simulink model "dc_motor"  (R2024a)
settings: Solver=VariableStepAuto  StartTime=0.0  StopTime=10.0  RelTol=1e-3
values from neighbouring files (symbols this model uses):
  b = 50    [my_cruise_bode.m]    (also in my_cruise_digital.m; my_cruise_lag.m; my_cruise_pid.m; my_cruise_rlocus.m)
  J = 0.01    [my_motor_rlocus.m]    (also in my_motor_v_bode.m; my_motor_v_cl.m; my_motor_v_tf.m)
  K = 0.01    [my_motor_rlocus.m]    (also in my_motor_v_bode.m; my_motor_v_cl.m; my_motor_v_tf.m)
  L = 0.5    [my_motor_rlocus.m]    (also in my_motor_v_bode.m; my_motor_v_cl.m; my_motor_v_tf.m)
  R = 1    [my_motor_rlocus.m]    (also in my_motor_v_bode.m; my_motor_v_cl.m; my_motor_v_tf.m)
settings Model: Creator=user  LastModifiedBy=user

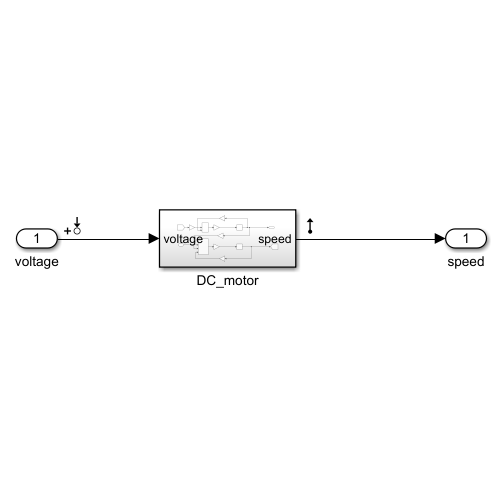
[thumbnail: Simulink's stored preview of the top-level diagram]
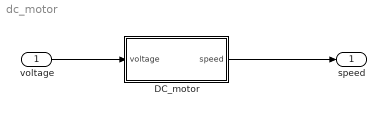
== system dc_motor ==
  voltage : Inport
  DC_motor : Subsystem
  speed : Outport
  wires:
  voltage/1 -> DC_motor/1(voltage)
  DC_motor/1(speed) -> speed/1

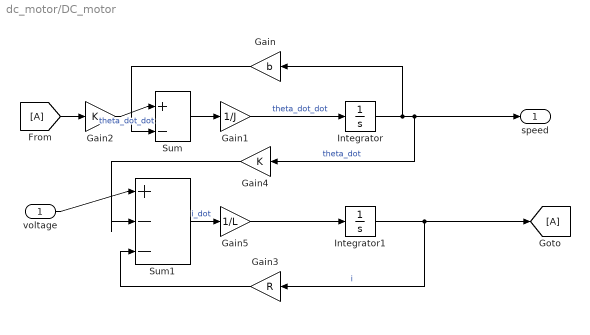
== system dc_motor/DC_motor ==
  voltage : Inport
  From : From
  Gain : Gain  Gain=b
  Gain1 : Gain  Gain=1/J
  Gain2 : Gain  Gain=K
  Gain3 : Gain  Gain=R
  Gain4 : Gain  Gain=K
  Gain5 : Gain  Gain=1/L
  Goto : Goto
  Integrator : Integrator
  Integrator1 : Integrator
  Sum : Sum  Inputs=|+-
  Sum1 : Sum  Inputs=|+--
  speed : Outport
  wires:
  Gain5/1 -> Integrator1/1
  From/1 -> Gain2/1
  Integrator1/1 -> Gain3/1, Goto/1  "i"
  Sum1/1 -> Gain5/1  "i_dot"
  Gain4/1 -> Sum1/2
  Sum/1 -> Gain1/1
  Gain1/1 -> Integrator/1  "theta_dot_dot"
  voltage/1 -> Sum1/1
  Gain2/1 -> Sum/1  "theta_dot_dot"
  Integrator/1 -> Gain/1, speed/1, Gain4/1  "theta_dot"
  Gain/1 -> Sum/2
  Gain3/1 -> Sum1/3
